simulink model "swim_12B_tmp"  (Simulink 9.0)
settings: Solver=FixedStepDiscrete  StartTime=0.0  StopTime=10.0  RelTol=1e-3  EnableMultiTasking=on
values from neighbouring files (symbols this model uses):
  E_DI_CATI = 0    [swim_12B_data.mat]
  E_DI_DOWN_OR_LOCKED = 0    [swim_12B_data.mat]
  E_DI_UP_AND_NORMAL = 1    [swim_12B_data.mat]
  E_MUX_ENABLED = 1    [swim_12B_data.mat]
  E_OLC_INTERLOCK_NOT_FAILED = 0    [swim_12B_data.mat]
  E_SWIM_ALLOWED = 1    [swim_12B_data.mat]
  E_SWIM_NOT_ALLOWED = 0    [swim_12B_data.mat]
  E_SWIM_WARNING_OFF = 0    [swim_12B_data.mat]
  E_SWIM_WARNING_ON = 1    [swim_12B_data.mat]
settings Model: Creator=belottr  LastModifiedBy=hbourbou
settings DataIOCC: LimitDataPoints=on
settings OptimizationCC: DefaultParameterBehavior=Inlined  ExpressionDepthLimit=2147483647
settings DebuggingCC: SolverPrmCheckMsg=warning  StateNameClashWarn=warning
settings ModelReferenceCC: UpdateModelReferenceTargets=IfOutOfDate
settings GRTTargetCC: GeneratePreprocessorConditionals=Disable all

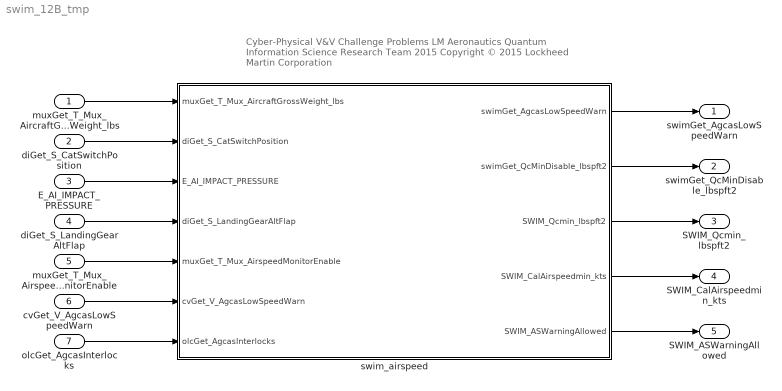
== system swim_12B_tmp ==
  note: Cyber-Physical V&V Challenge Problems
      | LM Aeronautics Quantum Information Science Research Team 2015
      | Copyright © 2015 Lockheed Martin Corporation
  muxGet_T_Mux_AircraftGrossWeight_lbs : Inport  OutDataTypeStr=double
  diGet_S_CatSwitchPosition : Inport  Port=2  OutDataTypeStr=int32
  E_AI_IMPACT_PRESSURE : Inport  Port=3  OutDataTypeStr=double
  diGet_S_LandingGearAltFlap : Inport  Port=4  OutDataTypeStr=boolean
  muxGet_T_Mux_AirspeedMonitorEnable : Inport  Port=5  OutDataTypeStr=boolean
  cvGet_V_AgcasLowSpeedWarn : Inport  Port=6  OutDataTypeStr=boolean
  olcGet_AgcasInterlocks : Inport  Port=7  OutDataTypeStr=boolean
  swim_airspeed : Subsystem
  swimGet_AgcasLowSpeedWarn : Outport  VectorParamsAs1DForOutWhenUnconnected=off
  swimGet_QcMinDisable_lbspft2 : Outport  Port=2  VectorParamsAs1DForOutWhenUnconnected=off
  SWIM_Qcmin_lbspft2 : Outport  Port=3  VectorParamsAs1DForOutWhenUnconnected=off
  SWIM_CalAirspeedmin_kts : Outport  Port=4  VectorParamsAs1DForOutWhenUnconnected=off
  SWIM_ASWarningAllowed : Outport  Port=5  VectorParamsAs1DForOutWhenUnconnected=off
  wires:
  muxGet_T_Mux_AircraftGrossWeight_lbs/1 -> swim_airspeed/1(muxGet_T_Mux_AircraftGrossWeight_lbs)
  diGet_S_CatSwitchPosition/1 -> swim_airspeed/2(diGet_S_CatSwitchPosition)
  E_AI_IMPACT_PRESSURE/1 -> swim_airspeed/3(E_AI_IMPACT_PRESSURE)
  diGet_S_LandingGearAltFlap/1 -> swim_airspeed/4(diGet_S_LandingGearAltFlap)
  muxGet_T_Mux_AirspeedMonitorEnable/1 -> swim_airspeed/5(muxGet_T_Mux_AirspeedMonitorEnable)
  cvGet_V_AgcasLowSpeedWarn/1 -> swim_airspeed/6(cvGet_V_AgcasLowSpeedWarn)
  olcGet_AgcasInterlocks/1 -> swim_airspeed/7(olcGet_AgcasInterlocks)
  swim_airspeed/3(SWIM_Qcmin_lbspft2) -> SWIM_Qcmin_lbspft2/1
  swim_airspeed/2(swimGet_QcMinDisable_lbspft2) -> swimGet_QcMinDisable_lbspft2/1
  swim_airspeed/1(swimGet_AgcasLowSpeedWarn) -> swimGet_AgcasLowSpeedWarn/1
  swim_airspeed/4(SWIM_CalAirspeedmin_kts) -> SWIM_CalAirspeedmin_kts/1
  swim_airspeed/5(SWIM_ASWarningAllowed) -> SWIM_ASWarningAllowed/1

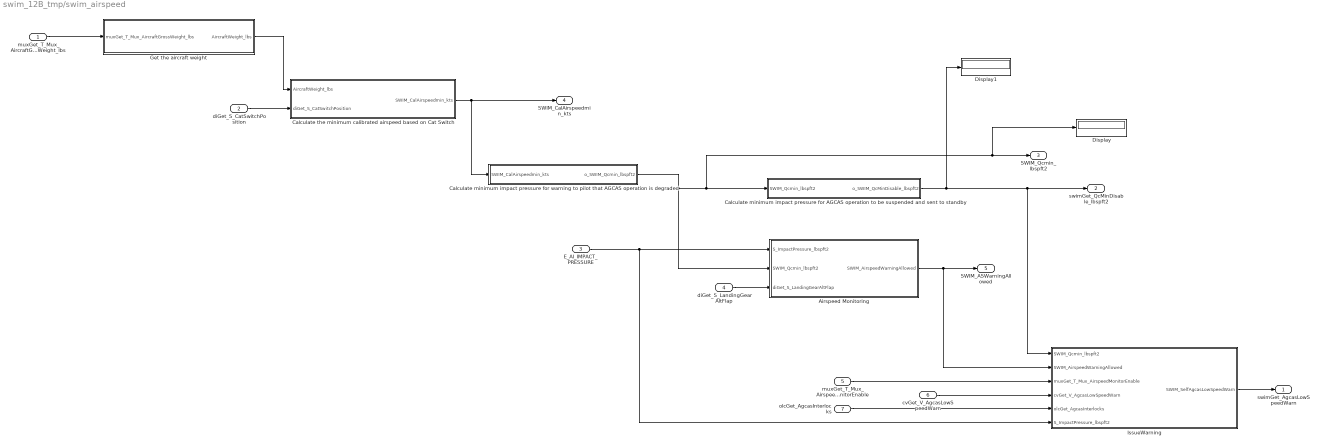
== system swim_12B_tmp/swim_airspeed ==
  muxGet_T_Mux_AircraftGrossWeight_lbs : Inport
  diGet_S_CatSwitchPosition : Inport  Port=2
  E_AI_IMPACT_PRESSURE : Inport  Port=3
  diGet_S_LandingGearAltFlap : Inport  Port=4
  muxGet_T_Mux_AirspeedMonitorEnable : Inport  Port=5
  cvGet_V_AgcasLowSpeedWarn : Inport  Port=6
  olcGet_AgcasInterlocks : Inport  Port=7
  Airspeed Monitoring : Subsystem
  Calculate minimum impact pressure for AGCAS operation to be suspended and sent to standby : Subsystem
  Calculate minimum impact pressure for warning to pilot that AGCAS operation is degraded : Subsystem
  Calculate the minimum calibrated airspeed based on Cat Switch : Subsystem
  Display : Display
  Display1 : Display
  Get the aircraft weight : Subsystem
  IssueWarning : Subsystem
  swimGet_AgcasLowSpeedWarn : Outport  VectorParamsAs1DForOutWhenUnconnected=off
  swimGet_QcMinDisable_lbspft2 : Outport  Port=2  VectorParamsAs1DForOutWhenUnconnected=off
  SWIM_Qcmin_lbspft2 : Outport  Port=3  VectorParamsAs1DForOutWhenUnconnected=off
  SWIM_CalAirspeedmin_kts : Outport  Port=4  VectorParamsAs1DForOutWhenUnconnected=off
  SWIM_ASWarningAllowed : Outport  Port=5  VectorParamsAs1DForOutWhenUnconnected=off
  wires:
  muxGet_T_Mux_AircraftGrossWeight_lbs/1 -> Get the aircraft weight/1(muxGet_T_Mux_AircraftGrossWeight_lbs)
  diGet_S_CatSwitchPosition/1 -> Calculate the minimum calibrated airspeed based on Cat Switch/2(diGet_S_CatSwitchPosition)
  Get the aircraft weight/1(AircraftWeight_lbs) -> Calculate the minimum calibrated airspeed based on Cat Switch/1(AircraftWeight_lbs)
  Calculate the minimum calibrated airspeed based on Cat Switch/1(SWIM_CalAirspeedmin_kts) -> Calculate minimum impact pressure for warning to pilot that AGCAS operation is degraded/1(SWIM_CalAirspeedmin_kts), SWIM_CalAirspeedmin_kts/1
  E_AI_IMPACT_PRESSURE/1 -> IssueWarning/6(S_ImpactPressure_lbspft2), Airspeed Monitoring/1(S_ImpactPressure_lbspft2)
  diGet_S_LandingGearAltFlap/1 -> Airspeed Monitoring/3(diGet_S_LandingGearAltFlap)
  IssueWarning/1(SWIM_SelfAgcasLowSpeedWarn) -> swimGet_AgcasLowSpeedWarn/1
  muxGet_T_Mux_AirspeedMonitorEnable/1 -> IssueWarning/3(muxGet_T_Mux_AirspeedMonitorEnable)
  cvGet_V_AgcasLowSpeedWarn/1 -> IssueWarning/4(cvGet_V_AgcasLowSpeedWarn)
  olcGet_AgcasInterlocks/1 -> IssueWarning/5(olcGet_AgcasInterlocks)
  Calculate minimum impact pressure for AGCAS operation to be suspended and sent to standby/1(o_SWIM_QcMinDisable_lbspft2) -> Display1/1, IssueWarning/1(SWIM_Qcmin_lbspft2), swimGet_QcMinDisable_lbspft2/1
  Airspeed Monitoring/1(SWIM_AirspeedWarningAllowed) -> IssueWarning/2(SWIM_AirspeedWarningAllowed), SWIM_ASWarningAllowed/1
  Calculate minimum impact pressure for warning to pilot that AGCAS operation is degraded/1(o_SWIM_Qcmin_lbspft2) -> Airspeed Monitoring/2(SWIM_Qcmin_lbspft2), Display/1, SWIM_Qcmin_lbspft2/1, Calculate minimum impact pressure for AGCAS operation to be suspended and sent to standby/1(SWIM_Qcmin_lbspft2)

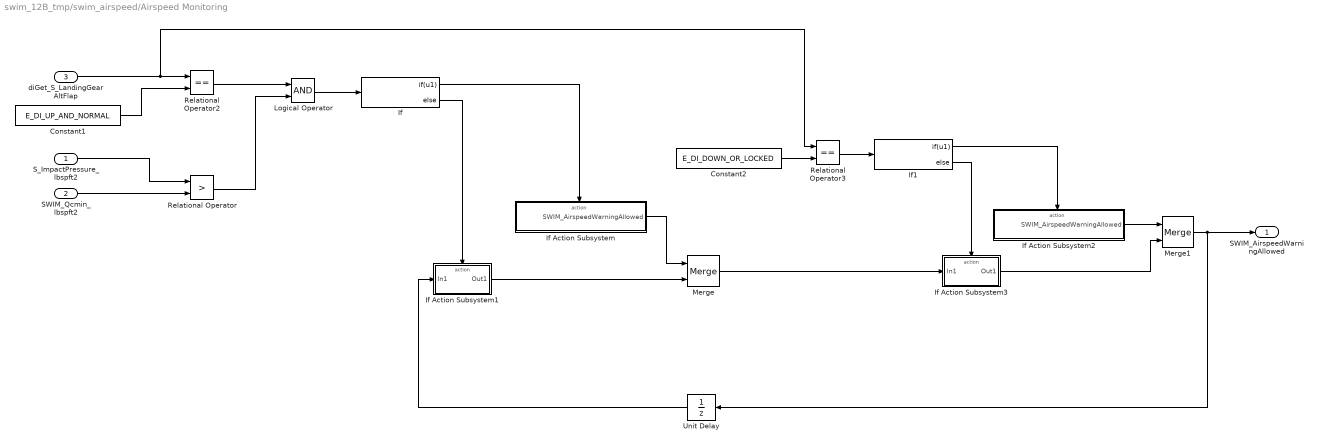
== system swim_12B_tmp/swim_airspeed/Airspeed Monitoring ==
  S_ImpactPressure_lbspft2 : Inport
  SWIM_Qcmin_lbspft2 : Inport  Port=2
  diGet_S_LandingGearAltFlap : Inport  Port=3
  Constant1 : Constant  Value=E_DI_UP_AND_NORMAL
  Constant2 : Constant  Value=E_DI_DOWN_OR_LOCKED
  If : If  IfExpression=u1
  If Action Subsystem : Subsystem  TreatAsAtomicUnit=on
  If Action Subsystem1 : Subsystem  TreatAsAtomicUnit=on
  If Action Subsystem2 : Subsystem  TreatAsAtomicUnit=on
  If Action Subsystem3 : Subsystem  TreatAsAtomicUnit=on
  If1 : If  IfExpression=u1
  Logical Operator : Logic  AllPortsSameDT=off  OutDataTypeStr=boolean
  Merge : Merge
  Merge1 : Merge
  Relational Operator : RelationalOperator  Operator=>  OutDataTypeStr=boolean  RndMeth=Nearest
  Relational Operator2 : RelationalOperator  Operator===  OutDataTypeStr=boolean  RndMeth=Nearest
  Relational Operator3 : RelationalOperator  Operator===  OutDataTypeStr=boolean  RndMeth=Nearest
  Unit Delay : UnitDelay  InitialCondition=E_SWIM_NOT_ALLOWED  SampleTime=-1  HasFrameUpgradeWarning=on
  SWIM_AirspeedWarningAllowed : Outport  VectorParamsAs1DForOutWhenUnconnected=off
  wires:
  S_ImpactPressure_lbspft2/1 -> Relational Operator/1
  SWIM_Qcmin_lbspft2/1 -> Relational Operator/2
  diGet_S_LandingGearAltFlap/1 -> Relational Operator3/1, Relational Operator2/1
  Constant1/1 -> Relational Operator2/2
  If/1 -> If Action Subsystem/Action
  If/2 -> If Action Subsystem1/Action
  If Action Subsystem/1(SWIM_AirspeedWarningAllowed) -> Merge/1
  If Action Subsystem1/1(Out1) -> Merge/2
  Constant2/1 -> Relational Operator3/2
  Relational Operator3/1 -> If1/1
  Relational Operator/1 -> Logical Operator/2
  Relational Operator2/1 -> Logical Operator/1
  Logical Operator/1 -> If/1
  If1/1 -> If Action Subsystem2/Action
  If1/2 -> If Action Subsystem3/Action
  If Action Subsystem2/1(SWIM_AirspeedWarningAllowed) -> Merge1/1
  If Action Subsystem3/1(Out1) -> Merge1/2
  Merge/1 -> If Action Subsystem3/1(In1)
  Merge1/1 -> Unit Delay/1, SWIM_AirspeedWarningAllowed/1
  Unit Delay/1 -> If Action Subsystem1/1(In1)

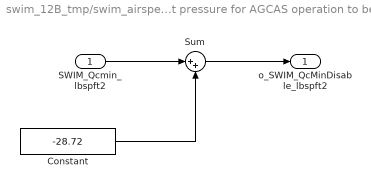
== system swim_12B_tmp/swim_airspeed/Calculate minimum impact pressure for AGCAS operation to be suspended and sent to standby ==
  SWIM_Qcmin_lbspft2 : Inport
  Constant : Constant  Value=-28.72
  Sum : Sum  Inputs=|++
  o_SWIM_QcMinDisable_lbspft2 : Outport  VectorParamsAs1DForOutWhenUnconnected=off
  wires:
  SWIM_Qcmin_lbspft2/1 -> Sum/1
  Constant/1 -> Sum/2
  Sum/1 -> o_SWIM_QcMinDisable_lbspft2/1

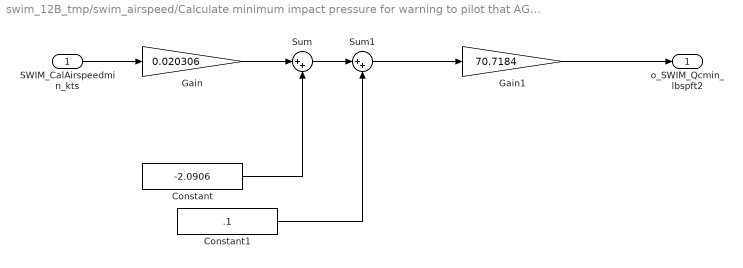
== system swim_12B_tmp/swim_airspeed/Calculate minimum impact pressure for warning to pilot that AGCAS operation is degraded ==
  SWIM_CalAirspeedmin_kts : Inport
  Constant : Constant  Value=-2.0906
  Constant1 : Constant  Value=.1
  Gain : Gain  Gain=0.020306
  Gain1 : Gain  Gain=70.7184
  Sum : Sum  Inputs=|++
  Sum1 : Sum  Inputs=|++
  o_SWIM_Qcmin_lbspft2 : Outport  VectorParamsAs1DForOutWhenUnconnected=off
  wires:
  SWIM_CalAirspeedmin_kts/1 -> Gain/1
  Gain/1 -> Sum/1
  Constant/1 -> Sum/2
  Sum/1 -> Sum1/1
  Constant1/1 -> Sum1/2
  Sum1/1 -> Gain1/1
  Gain1/1 -> o_SWIM_Qcmin_lbspft2/1

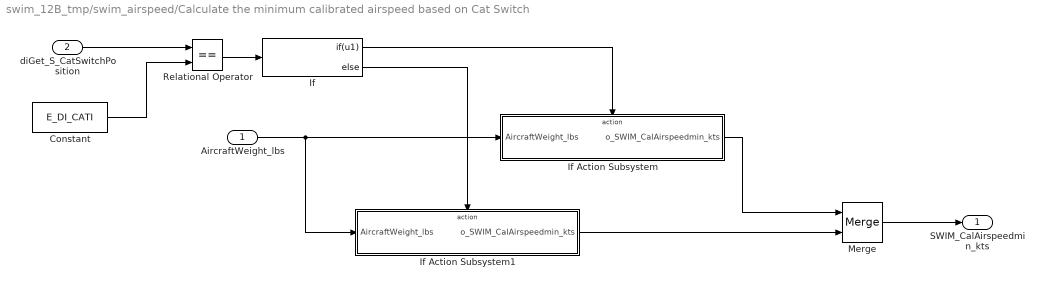
== system swim_12B_tmp/swim_airspeed/Calculate the minimum calibrated airspeed based on Cat Switch ==
  AircraftWeight_lbs : Inport
  diGet_S_CatSwitchPosition : Inport  Port=2
  Constant : Constant  Value=E_DI_CATI
  If : If  IfExpression=u1
  If Action Subsystem : Subsystem  TreatAsAtomicUnit=on
  If Action Subsystem1 : Subsystem  TreatAsAtomicUnit=on
  Merge : Merge
  Relational Operator : RelationalOperator  Operator===  OutDataTypeStr=boolean  RndMeth=Nearest
  SWIM_CalAirspeedmin_kts : Outport  VectorParamsAs1DForOutWhenUnconnected=off
  wires:
  If/1 -> If Action Subsystem/Action
  If/2 -> If Action Subsystem1/Action
  If Action Subsystem/1(o_SWIM_CalAirspeedmin_kts) -> Merge/1
  If Action Subsystem1/1(o_SWIM_CalAirspeedmin_kts) -> Merge/2
  Merge/1 -> SWIM_CalAirspeedmin_kts/1
  AircraftWeight_lbs/1 -> If Action Subsystem/1(AircraftWeight_lbs), If Action Subsystem1/1(AircraftWeight_lbs)
  Constant/1 -> Relational Operator/2
  diGet_S_CatSwitchPosition/1 -> Relational Operator/1
  Relational Operator/1 -> If/1

== system swim_12B_tmp/swim_airspeed/Get the aircraft weight ==
  muxGet_T_Mux_AircraftGrossWeight_lbs : Inport
  AircraftWeight_lbs : Outport  VectorParamsAs1DForOutWhenUnconnected=off
  wires:
  muxGet_T_Mux_AircraftGrossWeight_lbs/1 -> AircraftWeight_lbs/1

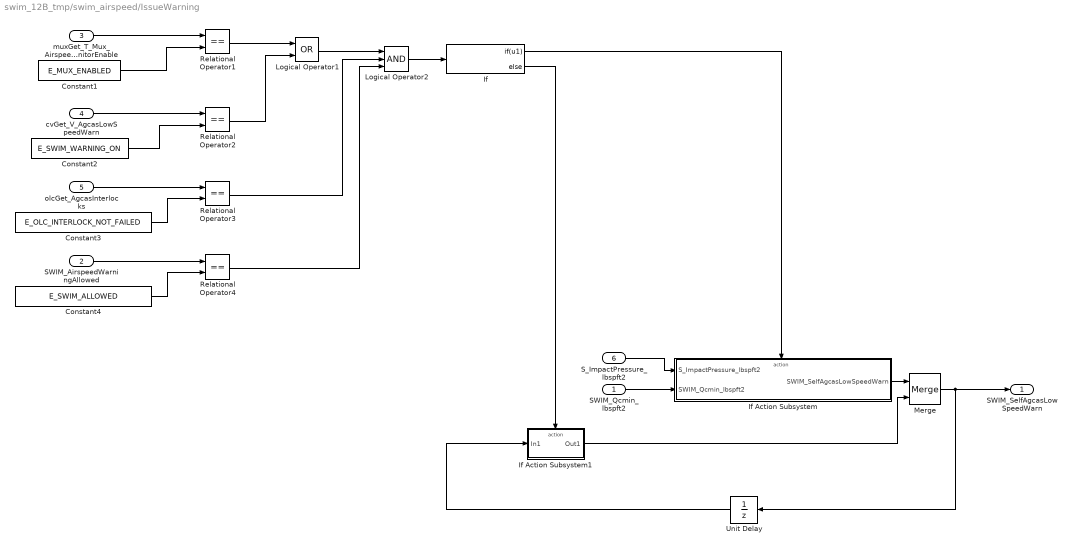
== system swim_12B_tmp/swim_airspeed/IssueWarning ==
  SWIM_Qcmin_lbspft2 : Inport
  SWIM_AirspeedWarningAllowed : Inport  Port=2
  muxGet_T_Mux_AirspeedMonitorEnable : Inport  Port=3
  cvGet_V_AgcasLowSpeedWarn : Inport  Port=4
  olcGet_AgcasInterlocks : Inport  Port=5
  S_ImpactPressure_lbspft2 : Inport  Port=6
  Constant1 : Constant  Value=E_MUX_ENABLED
  Constant2 : Constant  Value=E_SWIM_WARNING_ON
  Constant3 : Constant  Value=E_OLC_INTERLOCK_NOT_FAILED
  Constant4 : Constant  Value=E_SWIM_ALLOWED
  If : If  IfExpression=u1
  If Action Subsystem : Subsystem  TreatAsAtomicUnit=on
  If Action Subsystem1 : Subsystem  TreatAsAtomicUnit=on
  Logical Operator1 : Logic  Operator=OR  AllPortsSameDT=off  OutDataTypeStr=boolean
  Logical Operator2 : Logic  Inputs=3  AllPortsSameDT=off  OutDataTypeStr=boolean
  Merge : Merge
  Relational Operator{1..4} (4 alike) : RelationalOperator  Operator===  OutDataTypeStr=boolean  RndMeth=Nearest
  Unit Delay : UnitDelay  InitialCondition=E_SWIM_WARNING_OFF  SampleTime=-1  HasFrameUpgradeWarning=on
  SWIM_SelfAgcasLowSpeedWarn : Outport  VectorParamsAs1DForOutWhenUnconnected=off
  wires:
  muxGet_T_Mux_AirspeedMonitorEnable/1 -> Relational Operator1/1
  cvGet_V_AgcasLowSpeedWarn/1 -> Relational Operator2/1
  Constant2/1 -> Relational Operator2/2
  Constant1/1 -> Relational Operator1/2
  olcGet_AgcasInterlocks/1 -> Relational Operator3/1
  Constant3/1 -> Relational Operator3/2
  SWIM_AirspeedWarningAllowed/1 -> Relational Operator4/1
  Constant4/1 -> Relational Operator4/2
  Relational Operator1/1 -> Logical Operator1/1
  Relational Operator2/1 -> Logical Operator1/2
  Logical Operator1/1 -> Logical Operator2/1
  Relational Operator3/1 -> Logical Operator2/2
  Relational Operator4/1 -> Logical Operator2/3
  Logical Operator2/1 -> If/1
  If/1 -> If Action Subsystem/Action
  If/2 -> If Action Subsystem1/Action
  SWIM_Qcmin_lbspft2/1 -> If Action Subsystem/2(SWIM_Qcmin_lbspft2)
  If Action Subsystem/1(SWIM_SelfAgcasLowSpeedWarn) -> Merge/1
  Merge/1 -> Unit Delay/1, SWIM_SelfAgcasLowSpeedWarn/1
  If Action Subsystem1/1(Out1) -> Merge/2
  Unit Delay/1 -> If Action Subsystem1/1(In1)
  S_ImpactPressure_lbspft2/1 -> If Action Subsystem/1(S_ImpactPressure_lbspft2)

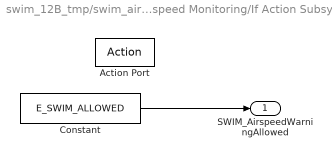
== system swim_12B_tmp/swim_airspeed/Airspeed Monitoring/If Action Subsystem ==
  Action Port : ActionPort
  Constant : Constant  Value=E_SWIM_ALLOWED
  SWIM_AirspeedWarningAllowed : Outport  VectorParamsAs1DForOutWhenUnconnected=off
  wires:
  Constant/1 -> SWIM_AirspeedWarningAllowed/1

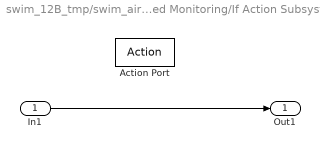
== system swim_12B_tmp/swim_airspeed/Airspeed Monitoring/If Action Subsystem1 ==
  In1 : Inport
  Action Port : ActionPort
  Out1 : Outport  VectorParamsAs1DForOutWhenUnconnected=off
  wires:
  In1/1 -> Out1/1

== system swim_12B_tmp/swim_airspeed/Airspeed Monitoring/If Action Subsystem2 ==
  Action Port : ActionPort
  Constant : Constant  Value=E_SWIM_NOT_ALLOWED
  SWIM_AirspeedWarningAllowed : Outport  VectorParamsAs1DForOutWhenUnconnected=off
  wires:
  Constant/1 -> SWIM_AirspeedWarningAllowed/1

== system swim_12B_tmp/swim_airspeed/Airspeed Monitoring/If Action Subsystem3 ==
  In1 : Inport
  Action Port : ActionPort
  Out1 : Outport  VectorParamsAs1DForOutWhenUnconnected=off
  wires:
  In1/1 -> Out1/1

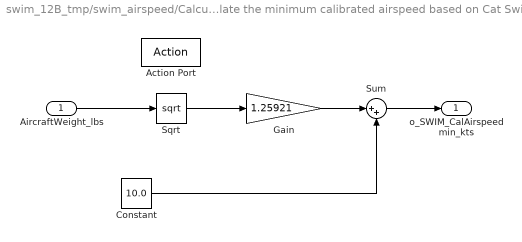
== system swim_12B_tmp/swim_airspeed/Calculate the minimum calibrated airspeed based on Cat Switch/If Action Subsystem ==
  AircraftWeight_lbs : Inport
  Action Port : ActionPort
  Constant : Constant  Value=10.0
  Gain : Gain  Gain=1.25921
  Sqrt : Sqrt  SaturateOnIntegerOverflow=on
  Sum : Sum  Inputs=|++
  o_SWIM_CalAirspeedmin_kts : Outport  VectorParamsAs1DForOutWhenUnconnected=off
  wires:
  AircraftWeight_lbs/1 -> Sqrt/1
  Gain/1 -> Sum/1
  Constant/1 -> Sum/2
  Sum/1 -> o_SWIM_CalAirspeedmin_kts/1
  Sqrt/1 -> Gain/1

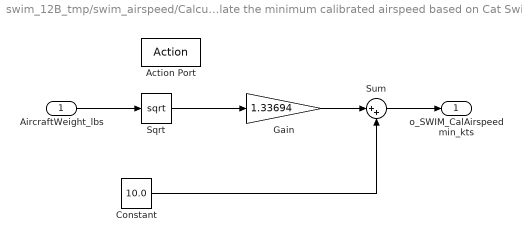
== system swim_12B_tmp/swim_airspeed/Calculate the minimum calibrated airspeed based on Cat Switch/If Action Subsystem1 ==
  AircraftWeight_lbs : Inport
  Action Port : ActionPort
  Constant : Constant  Value=10.0
  Gain : Gain  Gain=1.33694
  Sqrt : Sqrt  SaturateOnIntegerOverflow=on
  Sum : Sum  Inputs=|++
  o_SWIM_CalAirspeedmin_kts : Outport  VectorParamsAs1DForOutWhenUnconnected=off
  wires:
  Sum/1 -> o_SWIM_CalAirspeedmin_kts/1
  Constant/1 -> Sum/2
  Gain/1 -> Sum/1
  AircraftWeight_lbs/1 -> Sqrt/1
  Sqrt/1 -> Gain/1

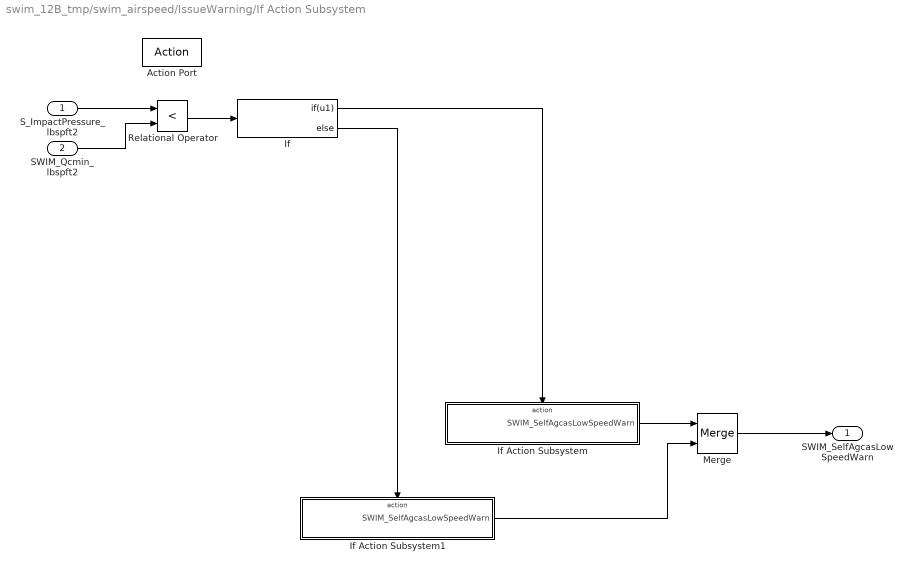
== system swim_12B_tmp/swim_airspeed/IssueWarning/If Action Subsystem ==
  S_ImpactPressure_lbspft2 : Inport
  SWIM_Qcmin_lbspft2 : Inport  Port=2
  Action Port : ActionPort
  If : If  IfExpression=u1
  If Action Subsystem : Subsystem  TreatAsAtomicUnit=on
  If Action Subsystem1 : Subsystem  TreatAsAtomicUnit=on
  Merge : Merge
  Relational Operator : RelationalOperator  Operator=<  OutDataTypeStr=boolean  RndMeth=Nearest
  SWIM_SelfAgcasLowSpeedWarn : Outport  VectorParamsAs1DForOutWhenUnconnected=off
  wires:
  S_ImpactPressure_lbspft2/1 -> Relational Operator/1
  SWIM_Qcmin_lbspft2/1 -> Relational Operator/2
  If/1 -> If Action Subsystem/Action
  Relational Operator/1 -> If/1
  Merge/1 -> SWIM_SelfAgcasLowSpeedWarn/1
  If Action Subsystem/1(SWIM_SelfAgcasLowSpeedWarn) -> Merge/1
  If Action Subsystem1/1(SWIM_SelfAgcasLowSpeedWarn) -> Merge/2
  If/2 -> If Action Subsystem1/Action

== system swim_12B_tmp/swim_airspeed/IssueWarning/If Action Subsystem1 ==
  In1 : Inport
  Action Port : ActionPort
  Out1 : Outport  VectorParamsAs1DForOutWhenUnconnected=off
  wires:
  In1/1 -> Out1/1

== system swim_12B_tmp/swim_airspeed/IssueWarning/If Action Subsystem/If Action Subsystem ==
  Action Port : ActionPort
  Constant : Constant  Value=E_SWIM_WARNING_ON
  SWIM_SelfAgcasLowSpeedWarn : Outport  VectorParamsAs1DForOutWhenUnconnected=off
  wires:
  Constant/1 -> SWIM_SelfAgcasLowSpeedWarn/1

== system swim_12B_tmp/swim_airspeed/IssueWarning/If Action Subsystem/If Action Subsystem1 ==
  Action Port : ActionPort
  Constant : Constant  Value=E_SWIM_WARNING_OFF
  SWIM_SelfAgcasLowSpeedWarn : Outport  VectorParamsAs1DForOutWhenUnconnected=off
  wires:
  Constant/1 -> SWIM_SelfAgcasLowSpeedWarn/1
